simulink model "BCM2_4"  (R2021b)
settings: Solver=FixedStepDiscrete  StartTime=0.0  StopTime=1  FixedStep=0.001  RelTol=1e-3  EnableMultiTasking=on
InitFcn:
  | mbd_mpc_consistency_checks(bdroot(gcs));
model workspace (MAT data in the model file):
  CAN_rec = Simulink.Signal
  CAN_rec.DataType = 'Bus: CAN_receive'
  CAN_rec.Dimensions = 1
  CAN_rec.DimensionsMode = 'auto'
  CAN_rec.Complexity = 'auto'
  CAN_rec.SampleTime = -1
  CAN_rec.SamplingMode = 'auto'
  CAN_transm_stat = Simulink.Signal
  CAN_transm_stat.DataType = 'boolean'
  CAN_transm_stat.Dimensions = 64
  CAN_transm_stat.DimensionsMode = 'auto'
  CAN_transm_stat.Complexity = 'auto'
  CAN_transm_stat.SampleTime = -1
  CAN_transm_stat.SamplingMode = 'auto'
  CAN_trm = Simulink.Signal
  CAN_trm.DataType = 'Bus: CAN_transmit'
  CAN_trm.Dimensions = 1
  CAN_trm.DimensionsMode = 'auto'
  CAN_trm.Complexity = 'auto'
  CAN_trm.SampleTime = -1
  CAN_trm.SamplingMode = 'auto'
  DITHER_CFB0 = Simulink.Parameter
  DITHER_CFB0.DataType = 'uint32'
  DITHER_CFB0.Complexity = 'real'
  DITHER_CFB0.Dimensions = [0 0]
  DITHER_CFB1 = Simulink.Parameter
  DITHER_CFB1.DataType = 'uint32'
  DITHER_CFB1.Complexity = 'real'
  DITHER_CFB1.Dimensions = [0 0]
  DITHER_CFB2 = Simulink.Parameter
  DITHER_CFB2.DataType = 'uint32'
  DITHER_CFB2.Complexity = 'real'
  DITHER_CFB2.Dimensions = [0 0]
  DITHER_EN0 = Simulink.Parameter
  DITHER_EN0.DataType = 'uint32'
  DITHER_EN0.Complexity = 'real'
  DITHER_EN0.Dimensions = [0 0]
  DITHER_EN1 = Simulink.Parameter
  DITHER_EN1.DataType = 'uint32'
  DITHER_EN1.Complexity = 'real'
  DITHER_EN1.Dimensions = [0 0]
  DITHER_EN2 = Simulink.Parameter
  DITHER_EN2.DataType = 'uint32'
  DITHER_EN2.Complexity = 'real'
  DITHER_EN2.Dimensions = [0 0]
  DITHER_SIZE0 = Simulink.Parameter
  DITHER_SIZE0.DataType = 'uint32'
  DITHER_SIZE0.Complexity = 'real'
  DITHER_SIZE0.Dimensions = [0 0]
  DITHER_SIZE1 = Simulink.Parameter
  DITHER_SIZE1.DataType = 'uint32'
  DITHER_SIZE1.Complexity = 'real'
  DITHER_SIZE1.Dimensions = [0 0]
  DITHER_SIZE2 = Simulink.Parameter
  DITHER_SIZE2.DataType = 'uint32'
  DITHER_SIZE2.Complexity = 'real'
  DITHER_SIZE2.Dimensions = [0 0]
  DITHER_STEP0 = Simulink.Parameter
  DITHER_STEP0.DataType = 'uint32'
  DITHER_STEP0.Complexity = 'real'
  DITHER_STEP0.Dimensions = [0 0]
  DITHER_STEP1 = Simulink.Parameter
  DITHER_STEP1.DataType = 'uint32'
  DITHER_STEP1.Complexity = 'real'
  DITHER_STEP1.Dimensions = [0 0]
  DITHER_STEP2 = Simulink.Parameter
  DITHER_STEP2.DataType = 'uint32'
  DITHER_STEP2.Complexity = 'real'
  DITHER_STEP2.Dimensions = [0 0]
  DITHER_SYNC0 = Simulink.Parameter
  DITHER_SYNC0.DataType = 'uint32'
  DITHER_SYNC0.Complexity = 'real'
  DITHER_SYNC0.Dimensions = [0 0]
  DITHER_SYNC1 = Simulink.Parameter
  DITHER_SYNC1.DataType = 'uint32'
  DITHER_SYNC1.Complexity = 'real'
  DITHER_SYNC1.Dimensions = [0 0]
  DITHER_SYNC2 = Simulink.Parameter
  DITHER_SYNC2.DataType = 'uint32'
  DITHER_SYNC2.Complexity = 'real'
  DITHER_SYNC2.Dimensions = [0 0]
  ECUMbut = Simulink.Signal
  ECUMbut.DataType = 'Bus: Ecumaster_buttons'
  ECUMbut.Dimensions = 1
  ECUMbut.DimensionsMode = 'Fixed'
  ECUMbut.Complexity = 'real'
  ECUMbut.SampleTime = -1
  ECUMbut.SamplingMode = 'auto'
  FAULTN = Simulink.Signal
  FAULTN.DataType = 'boolean'
  FAULTN.Dimensions = 1
  FAULTN.DimensionsMode = 'Fixed'
  FAULTN.Complexity = 'real'
  FAULTN.SampleTime = -1
  FAULTN.SamplingMode = 'auto'
  FAULTN.InitialValue = 'false'
  FM0 = Simulink.Parameter
  FM0.DataType = 'uint32'
  FM0.Complexity = 'real'
  FM0.Dimensions = [0 0]
  FM1 = Simulink.Parameter
  FM1.DataType = 'uint32'
  FM1.Complexity = 'real'
  FM1.Dimensions = [0 0]
  FM2 = Simulink.Parameter
  FM2.DataType = 'uint32'
  FM2.Complexity = 'real'
  FM2.Dimensions = [0 0]
  FME = Simulink.Parameter
  FME.DataType = 'uint32'
  FME.Complexity = 'real'
  FME.Dimensions = [0 0]
  Fsys_M = Simulink.Parameter
  Fsys_M.DataType = 'uint32'
  Fsys_M.Complexity = 'real'
  Fsys_M.Dimensions = [0 0]
  Fsys_N = Simulink.Parameter
  Fsys_N.DataType = 'uint32'
  Fsys_N.Complexity = 'real'
  Fsys_N.Dimensions = [0 0]
  Fsys_WDEN = Simulink.Parameter
  Fsys_WDEN.DataType = 'uint32'
  Fsys_WDEN.Complexity = 'real'
  Fsys_WDEN.Dimensions = [0 0]
  Fsys_div = Simulink.Parameter
  Fsys_div.DataType = 'uint32'
  Fsys_div.Complexity = 'real'
  Fsys_div.Dimensions = [0 0]
  HL0 = Simulink.Parameter
  HL0.DataType = 'uint32'
  HL0.Complexity = 'real'
  HL0.Dimensions = [0 0]
  HL1 = Simulink.Parameter
  HL1.DataType = 'uint32'
  HL1.Complexity = 'real'
  HL1.Dimensions = [0 0]
  HL2 = Simulink.Parameter
  HL2.DataType = 'uint32'
  HL2.Complexity = 'real'
  HL2.Dimensions = [0 0]
  IDIAG0 = Simulink.Parameter
  IDIAG0.DataType = 'uint32'
  IDIAG0.Complexity = 'real'
  IDIAG0.Dimensions = [0 0]
  IDIAG1 = Simulink.Parameter
  IDIAG1.DataType = 'uint32'
  IDIAG1.Complexity = 'real'
  IDIAG1.Dimensions = [0 0]
  IDIAG2 = Simulink.Parameter
  IDIAG2.DataType = 'uint32'
  IDIAG2.Complexity = 'real'
  IDIAG2.Dimensions = [0 0]
  Ivalve = Simulink.Signal
  Ivalve.DataType = 'uint16'
  Ivalve.Dimensions = 3
  Ivalve.DimensionsMode = 'Fixed'
  Ivalve.Complexity = 'real'
  Ivalve.SampleTime = -1
  Ivalve.SamplingMode = 'auto'
  KI_index0 = Simulink.Parameter
  KI_index0.DataType = 'uint32'
  KI_index0.Complexity = 'real'
  KI_index0.Dimensions = [0 0]
  KI_index1 = Simulink.Parameter
  KI_index1.DataType = 'uint32'
  KI_index1.Complexity = 'real'
  KI_index1.Dimensions = [0 0]
  KI_index2 = Simulink.Parameter
  KI_index2.DataType = 'uint32'
  KI_index2.Complexity = 'real'
  KI_index2.Dimensions = [0 0]
  PWM_Period0 = Simulink.Parameter
  PWM_Period0.DataType = 'uint32'
  PWM_Period0.Complexity = 'real'
  PWM_Period0.Dimensions = [0 0]
  PWM_Period1 = Simulink.Parameter
  PWM_Period1.DataType = 'uint32'
  PWM_Period1.Complexity = 'real'
  PWM_Period1.Dimensions = [0 0]
  PWM_Period2 = Simulink.Parameter
  PWM_Period2.DataType = 'uint32'
  PWM_Period2.Complexity = 'real'
  PWM_Period2.Dimensions = [0 0]
  RESN = Simulink.Signal
  RESN.DataType = 'boolean'
  RESN.Dimensions = 1
  RESN.DimensionsMode = 'Fixed'
  RESN.Complexity = 'real'
  RESN.SampleTime = -1
  RESN.SamplingMode = 'auto'
  RESN.InitialValue = 'false'
  SR0 = Simulink.Parameter
  SR0.DataType = 'uint32'
  SR0.Complexity = 'real'
  SR0.Dimensions = [0 0]
  SR1 = Simulink.Parameter
  SR1.DataType = 'uint32'
  SR1.Complexity = 'real'
  SR1.Dimensions = [0 0]
  SR2 = Simulink.Parameter
  SR2.DataType = 'uint32'
  SR2.Complexity = 'real'
  SR2.Dimensions = [0 0]
  Vparam = Simulink.Signal
  Vparam.DataType = 'Bus: Vparameters'
  Vparam.Dimensions = 1
  Vparam.DimensionsMode = 'Fixed'
  Vparam.Complexity = 'real'
  Vparam.SampleTime = -1
  Vparam.SamplingMode = 'auto'
  block_tle = Simulink.Signal
  block_tle.DataType = 'boolean'
  block_tle.Dimensions = 4
  block_tle.DimensionsMode = 'auto'
  block_tle.Complexity = 'real'
  block_tle.SampleTime = -1
  block_tle.SamplingMode = 'auto'
  disp = Simulink.Signal
  disp.DataType = 'Bus: display'
  disp.Dimensions = 1
  disp.DimensionsMode = 'auto'
  disp.Complexity = 'auto'
  disp.SampleTime = -1
  disp.SamplingMode = 'auto'
  ee_adr = Simulink.Signal
  ee_adr.DataType = 'uint8'
  ee_adr.Dimensions = 1
  ee_adr.DimensionsMode = 'auto'
  ee_adr.Complexity = 'real'
  ee_adr.SampleTime = -1
  ee_adr.SamplingMode = 'auto'
  ee_en_rd = Simulink.Signal
  ee_en_rd.DataType = 'boolean'
  ee_en_rd.Dimensions = 1
  ee_en_rd.DimensionsMode = 'auto'
  ee_en_rd.Complexity = 'real'
  ee_en_rd.SampleTime = -1
  ee_en_rd.SamplingMode = 'auto'
  ee_en_wr = Simulink.Signal
  ee_en_wr.DataType = 'boolean'
  ee_en_wr.Dimensions = 1
  ee_en_wr.DimensionsMode = 'auto'
  ee_en_wr.Complexity = 'real'
  ee_en_wr.SampleTime = -1
  ee_en_wr.SamplingMode = 'auto'
  ee_idle = Simulink.Signal
  ee_idle.DataType = 'boolean'
  ee_idle.Dimensions = 1
  ee_idle.DimensionsMode = 'auto'
  ee_idle.Complexity = 'real'
  ee_idle.SampleTime = -1
  ee_idle.SamplingMode = 'auto'
  ee_read = Simulink.Signal
  ee_read.DataType = 'uint16'
  ee_read.Dimensions = 1
  ee_read.DimensionsMode = 'auto'
  ee_read.Complexity = 'real'
  ee_read.SampleTime = -1
  ee_read.SamplingMode = 'auto'
  ee_recv = Simulink.Signal
  ee_recv.DataType = 'uint8'
  ee_recv.Dimensions = [1 5]
  ee_recv.DimensionsMode = 'auto'
  ee_recv.Complexity = 'real'
  ee_recv.SampleTime = -1
  ee_recv.SamplingMode = 'auto'
  ee_send = Simulink.Signal
  ee_send.DataType = 'uint16'
  ee_send.Dimensions = 1
  ee_send.DimensionsMode = 'auto'
  ee_send.Complexity = 'real'
  ee_send.SampleTime = -1
  ee_send.SamplingMode = 'auto'
  in_stats = Simulink.Signal
  in_stats.DataType = 'Bus: inputs_stat'
  in_stats.Dimensions = 1
  in_stats.DimensionsMode = 'Fixed'
  in_stats.Complexity = 'real'
  in_stats.SampleTime = -1
  in_stats.SamplingMode = 'auto'
  inputs = Simulink.Signal
  inputs.DataType = 'boolean'
  inputs.Dimensions = 44
  inputs.DimensionsMode = 'Fixed'
  inputs.Complexity = 'real'
  inputs.SampleTime = -1
  inputs.SamplingMode = 'auto'
  light = Simulink.Signal
  light.DataType = 'Bus: light_outs'
  light.Dimensions = 1
  light.DimensionsMode = 'Fixed'
  light.Complexity = 'real'
  light.SampleTime = -1
  light.SamplingMode = 'auto'
  out_drv = Simulink.Signal
  out_drv.DataType = 'boolean'
  out_drv.Dimensions = 16
  out_drv.DimensionsMode = 'Fixed'
  out_drv.Complexity = 'real'
  out_drv.SampleTime = -1
  out_drv.SamplingMode = 'auto'
  out_drv_test = Simulink.Signal
  out_drv_test.DataType = 'boolean'
  out_drv_test.Dimensions = 16
  out_drv_test.DimensionsMode = 'Fixed'
  out_drv_test.Complexity = 'real'
  out_drv_test.SampleTime = -1
  out_drv_test.SamplingMode = 'auto'
  out_test_en = Simulink.Signal
  out_test_en.DataType = 'boolean'
  out_test_en.Dimensions = 1
  out_test_en.DimensionsMode = 'Fixed'
  out_test_en.Complexity = 'real'
  out_test_en.SampleTime = -1
  out_test_en.SamplingMode = 'auto'
  recv_spi2 = Simulink.Signal
  recv_spi2.DataType = 'uint8'
  recv_spi2.Dimensions = 8
  recv_spi2.DimensionsMode = 'Fixed'
  recv_spi2.Complexity = 'real'
  recv_spi2.SampleTime = -1
  recv_spi2.SamplingMode = 'auto'
  ret = Simulink.Signal
  ret.DataType = 'Bus: retarder'
  ret.Dimensions = 1
  ret.DimensionsMode = 'Fixed'
  ret.Complexity = 'real'
  ret.SampleTime = -1
  ret.SamplingMode = 'auto'
  spi_rcv_tle82453 = Simulink.Signal
  spi_rcv_tle82453.DataType = 'uint8'
  spi_rcv_tle82453.Dimensions = [1 4]
  spi_rcv_tle82453.DimensionsMode = 'auto'
  spi_rcv_tle82453.Complexity = 'real'
  spi_rcv_tle82453.SampleTime = -1
  spi_rcv_tle82453.SamplingMode = 'auto'
  tle82453_Ivlv = Simulink.Signal
  tle82453_Ivlv.DataType = 'uint8'
  tle82453_Ivlv.Dimensions = 3
  tle82453_Ivlv.DimensionsMode = 'auto'
  tle82453_Ivlv.Complexity = 'real'
  tle82453_Ivlv.SampleTime = -1
  tle82453_Ivlv.SamplingMode = 'auto'
  tle82453_Ivlv.InitialValue = '[0 0 0]'
  tle82453_err = Simulink.Signal
  tle82453_err.DataType = 'uint32'
  tle82453_err.Dimensions = 1
  tle82453_err.DimensionsMode = 'auto'
  tle82453_err.Complexity = 'real'
  tle82453_err.SampleTime = -1
  tle82453_err.SamplingMode = 'auto'
  tle82453_reset = Simulink.Signal
  tle82453_reset.DataType = 'boolean'
  tle82453_reset.Dimensions = 1
  tle82453_reset.DimensionsMode = 'Fixed'
  tle82453_reset.Complexity = 'real'
  tle82453_reset.SampleTime = -1
  tle82453_reset.SamplingMode = 'auto'
  tle82453_reset.InitialValue = '0'
  wtdg_CAN = Simulink.Signal
  wtdg_CAN.DataType = 'Bus: WTDG_CAN'
  wtdg_CAN.Dimensions = 1
  wtdg_CAN.DimensionsMode = 'auto'
  wtdg_CAN.Complexity = 'real'
  wtdg_CAN.SampleTime = -1
  wtdg_CAN.SamplingMode = 'auto'
undefined symbols (not defined in the file or in its folder): color, LQFP
libraries: simulink x68, mbd_mpc574x_ec_toolbox x50, canmsglib x42, hdlsllib x9, commutil2 x7, etargetslib x4
(part 1 of 6)
Description:
  | Блок управления BCM
  | В качестве драйвера входов используется MC33978
settings Model: Creator=Дешкин Е.А.  LastModifiedBy=km-gir
settings SolverCC: AlgebraicLoopSolver=TrustRegion  AutoInsertRateTranBlk=on
settings DataIOCC: ExternalInput=off  InitialState=off  LimitDataPoints=on  SaveFormat=Array  SaveOutput=off  SignalLogging=off  SaveTime=off  ReturnWorkspaceOutputs=off
settings OptimizationCC: DefaultParameterBehavior=Inlined  PassReuseOutputArgsAs=Individual arguments  LifeSpan=inf  EfficientTunableParamExpr=on
settings DebuggingCC: MergeDetectMultiDrivingBlocksExec=none  SolverPrmCheckMsg=warning  InheritedTsInSrcMsg=none  MultiTaskDSMMsg=none  SingleTaskRateTransMsg=error  ParameterTunabilityLossMsg=error  UnconnectedInputMsg=error  UnconnectedOutputMsg=error  UnconnectedLineMsg=error  AllowSymbolicDim=off  UnknownTsInhSupMsg=error  StateNameClashWarn=warning  SFUnexpectedBacktrackingDiag=warning  SFNoUnconditionalDefaultTransitionDiag=warning  SFMachineParentedDataDiag=warning  ArithmeticOperatorsInVariantConditions=warning
settings HardwareCC: ProdBitPerPointer=32  ProdBitPerSizeT=32  ProdBitPerPtrDiffT=32  ProdLargestAtomicInteger=Long  ProdLargestAtomicFloat=Double  ProdEndianess=BigEndian  ProdWordSize=32  ProdHWDeviceType=Motorola PowerPC
settings ModelReferenceCC: PropagateSignalLabelsOutOfModel=off
settings SFSimCC: SimUseLocalCustomCode=off  MATLABDynamicMemAlloc=off  CustomCodeUndefinedFunction=UseInterfaceOnly
settings RTWCC: Description=Model Based Design Toolbox MPC57xx Code Generation Target  SystemTargetFile=mbd_mpc574x.tlc  MakeCommand=mbd_mpc574x_make_rtw  TemplateMakefile=mbd_mpc574x.tmf  GenerateReport=on  RTWUseLocalCustomCode=off  IncludeHyperlinkInReport=on  LaunchReport=on  GenerateTraceInfo=on  GenerateTraceReport=on  GenerateTraceReportSl=on  GenerateTraceReportSf=on  GenerateTraceReportEml=on
settings CodeAppCC: ForceParamTrailComments=on  IgnoreCustomStorageClasses=off  OperatorAnnotations=on  SimulinkDataObjDesc=on  SFDataObjDesc=on  MATLABFcnDesc=on  InsertBlockDesc=on  StateflowObjectComments=on  MATLABSourceComments=on
settings STFCustomTargetCC: MultiwordLength=256  CombineOutputUpdateFcns=on  ERTCustomFileBanners=on  SupportContinuousTime=off  SupportNonInlinedSFcns=off  RemoveResetFunc=on  MATLABClassNameForMDSCustomization=Simulink.SoftwareTarget.ERTCustomization  GRTInterface=off  SystemTargetFile=mbd_mpc574x.tlc
settings ERTTargetCC: ParMdlRefBuildCompliant=off  CompOptLevelCompliant=off  ConcurrentExecutionCompliant=off  ModelStepFunctionPrototypeControlCompliant=off  CPPClassGenCompliant=off  UseToolchainInfoCompliant=off  InlinedParameterPlacement=NonHierarchical  ERTSrcFileBannerTemplate=mbd_ert_code_template.cgt  ERTHdrFileBannerTemplate=mbd_ert_code_template.cgt  ERTDataSrcFileTemplate=mbd_ert_code_template.cgt  ERTDataHdrFileTemplate=mbd_ert_code_template.cgt  ERTCustomFileTemplate=example_file_process.tlc
settings ConfigComp: CovMetricSettings=dw  CovSaveCumulativeToWorkspaceVar=on  CovSaveSingleToWorkspaceVar=on  CovExternalEMLEnable=off

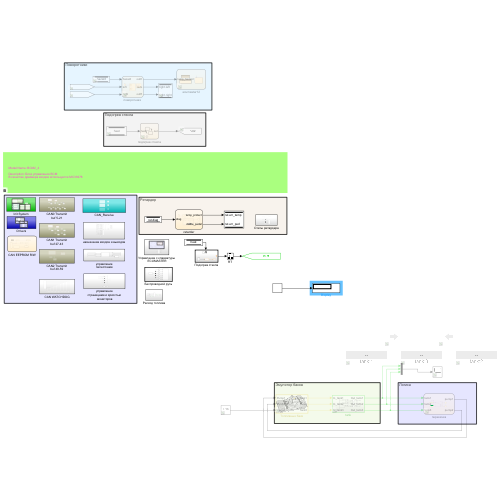
[thumbnail: Simulink's stored preview of the top-level diagram]
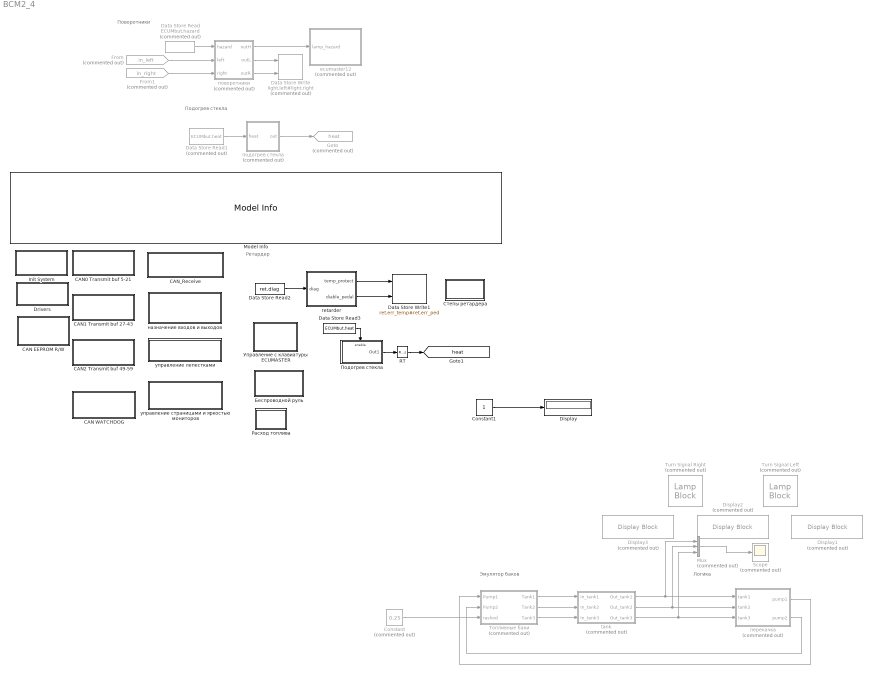
== system BCM2_4 ==
  note: Логика
  note: Эмулятор баков
  note: Подогрев стекла
  note: Поворотники
  note: Ретардер
  CAN EEPROM R/W : Stateflow chart  TreatAsAtomicUnit=on
  CAN WATCHDOG : Subsystem
  CAN0 Transmit buf 5-21 : Subsystem
  CAN1 Transmit buf 27-43 : Subsystem
  CAN2 Transmit buf 49-59 : Subsystem
  CAN_Receive : Subsystem  Priority=2
  Constant : Constant  Commented=on  Value=0.25
  Constant1 : Constant
  Data Store Read : DataStoreRead  Commented=on  DataStoreName=ECUMbut  DataStoreElements=ECUMbut.hazard  IndexOptions=Index vector (dialog)  Indices=1  OutputSizes=1
  Data Store Read1 : DataStoreRead  Commented=on  DataStoreName=ECUMbut  DataStoreElements=ECUMbut.heat  IndexOptions=Index vector (dialog)  Indices=1  OutputSizes=1
  Data Store Read2 : DataStoreRead  DataStoreName=ret  DataStoreElements=ret.diag  IndexOptions=Index vector (dialog)  Indices=1  OutputSizes=1
  Data Store Read3 : DataStoreRead  DataStoreName=ECUMbut  DataStoreElements=ECUMbut.heat  IndexOptions=Index vector (dialog)  Indices=1  OutputSizes=1
  Data Store Write : DataStoreWrite  Commented=on  DataStoreName=light  DataStoreElements=light.left#light.right  IndexOptions=Index vector (dialog)  Indices=1  OutputSizes=1
  Data Store Write1 : DataStoreWrite  DataStoreName=ret  DataStoreElements=ret.err_temp#ret.err_ped  IndexOptions=Index vector (dialog)  Indices=1  OutputSizes=1
  Display : Display
  Display1 : DisplayBlock  Commented=on  LabelPosition=Bottom  Format=short  Transparency=1
  Display2 : DisplayBlock  Commented=on  LabelPosition=Bottom  Format=short  Transparency=1
  Display3 : DisplayBlock  Commented=on  LabelPosition=Bottom  Format=short  Transparency=1
  Drivers : Subsystem
  From : From  Commented=on  GotoTag=in_left  TagVisibility=global
  From1 : From  Commented=on  GotoTag=in_right  TagVisibility=global
  Goto : Goto  Commented=on  GotoTag=heat  TagVisibility=global
  Init System : Subsystem
  Model Info : simulink/Model-Wide Utilities/Model Info  Frame=off  DisplayStringWithTags=|  HorizontalTextAlignment=Left  LeftAlignmentValue=0.02
      | Model Name: %<ModelName>
      | 
      | Description: %<Description>
  Mux : Mux  Commented=on  Inputs=3
  RT : RateTransition  OutPortSampleTime=0.01
  Scope : Scope  Commented=on
  Turn Signal Left : LampBlock  Commented=on  LabelPosition=Hide  Icon=TurnSignalLeft
  Turn Signal Right : LampBlock  Commented=on  LabelPosition=Hide  Icon=TurnSignalRight
  ecumaster12 : Stateflow chart  Commented=on  TreatAsAtomicUnit=on
  retarder : Stateflow chart  TreatAsAtomicUnit=on
  tank : Subsystem  Commented=on
  Беспроводной руль : Subsystem  TreatAsAtomicUnit=on  SystemSampleTime=0.01
  Подогрев стекла : Subsystem  TreatAsAtomicUnit=on
  Расход топлива : Subsystem
  Степы ретардера : Subsystem
  Топливные баки : Subsystem  Commented=on  TreatAsAtomicUnit=on  SystemSampleTime=1  mask{ft1=290, ft2=230, ft3=50}
      mask prompts: ft1 "Fuel tank1"; ft2 "Fuel tank2"; ft3 "Fuel tank3"
      mask Display: image('$imagefile'); % Use "Edit Image" on toolstrip to change.
  Управление с клавиатуры ECUMASTER : Subsystem
  назначение входов и выходов : Subsystem
  перекачка : Stateflow chart  Commented=on  TreatAsAtomicUnit=on
  поворотники : Stateflow chart  Commented=on  TreatAsAtomicUnit=on
  подогрев стекла : Stateflow chart  Commented=on  TreatAsAtomicUnit=on  mask{heat_off=3, heat_on=6}
      mask prompts: heat_off "Time OFF, minutes"; heat_on "Time ON, minutes"
  управление лепестками : Subsystem
  управление страницами и яркостью мониторов : Subsystem
  tag scope: heat=global
  wires:
  Data Store Read/1 -> поворотники/1(hazard)
  From/1 -> поворотники/2(left)
  From1/1 -> поворотники/3(right)
  поворотники/1(outH) -> ecumaster12/1(lamp_hazard)
  подогрев стекла/1(out) -> Goto/1
  поворотники/2(outL) -> Data Store Write/1
  поворотники/3(outR) -> Data Store Write/2
  retarder/2(" diable_pedal") -> Data Store Write1/2
  retarder/1(" temp_protect") -> Data Store Write1/1
  Data Store Read2/1 -> retarder/1(diag)
  Data Store Read1/1 -> подогрев стекла/1(heat)
  RT/1 -> [heat]
  Data Store Read3/1 -> Подогрев стекла/Enable
  Подогрев стекла/1(Out1) -> RT/1
  Топливные баки/1(Tank1) -> tank/1(In_tank1)
  Топливные баки/2(Tank2) -> tank/2(In_tank2)
  Топливные баки/3(Tank3) -> tank/3(In_tank3)
  tank/1(Out_tank1) -> Mux/1, перекачка/1(tank1)
  tank/2(Out_tank2) -> Mux/2, перекачка/2(tank2)
  tank/3(Out_tank3) -> Mux/3, перекачка/3(tank3)
  перекачка/2(pump2) -> Топливные баки/2(Pump2)
  Mux/1 -> Scope/1
  Constant/1 -> Топливные баки/3(rashod)
  перекачка/1(pump1) -> Топливные баки/1(Pump1)
  Constant1/1 -> Display/1

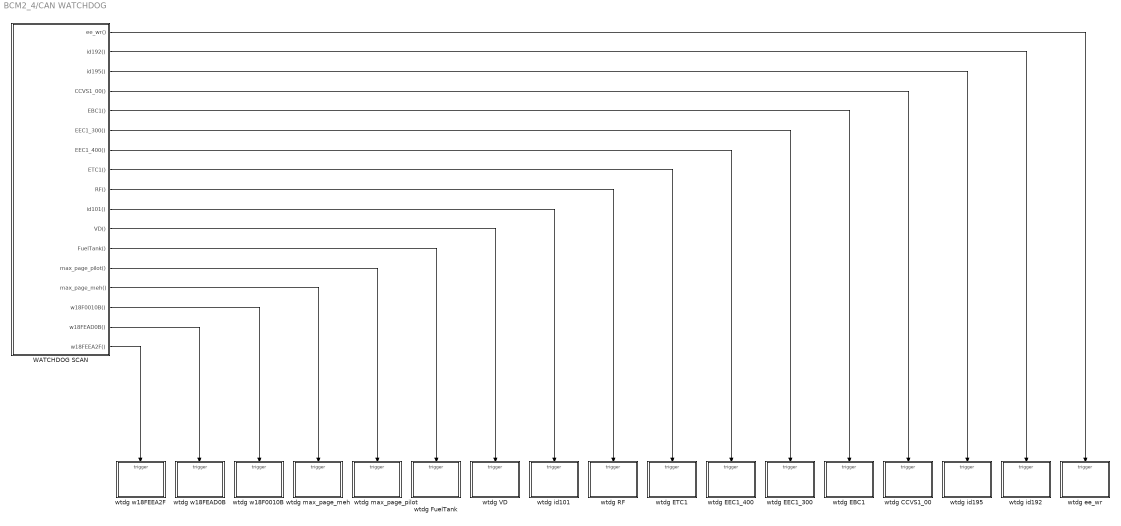
== system BCM2_4/CAN WATCHDOG ==
  WATCHDOG SCAN : Stateflow chart  TreatAsAtomicUnit=on
  wtdg CCVS1_00 : Subsystem  TreatAsAtomicUnit=on
  wtdg EBC1 : Subsystem  TreatAsAtomicUnit=on
  wtdg EEC1_300 : Subsystem  TreatAsAtomicUnit=on
  wtdg EEC1_400 : Subsystem  TreatAsAtomicUnit=on
  wtdg ETC1 : Subsystem  TreatAsAtomicUnit=on
  wtdg FuelTank : Subsystem  TreatAsAtomicUnit=on
  wtdg RF : Subsystem  TreatAsAtomicUnit=on
  wtdg VD : Subsystem  TreatAsAtomicUnit=on
  wtdg ee_wr : Subsystem  TreatAsAtomicUnit=on
  wtdg id101 : Subsystem  TreatAsAtomicUnit=on
  wtdg id192 : Subsystem  TreatAsAtomicUnit=on
  wtdg id195 : Subsystem  TreatAsAtomicUnit=on
  wtdg max_page_meh : Subsystem  TreatAsAtomicUnit=on
  wtdg max_page_pilot : Subsystem  TreatAsAtomicUnit=on
  wtdg w18F0010B : Subsystem  TreatAsAtomicUnit=on
  wtdg w18FEAD0B : Subsystem  TreatAsAtomicUnit=on
  wtdg w18FEEA2F : Subsystem  TreatAsAtomicUnit=on
  wires:
  WATCHDOG SCAN/9(RF()) -> wtdg RF/Trigger
  WATCHDOG SCAN/8(ETC1()) -> wtdg ETC1/Trigger
  WATCHDOG SCAN/7(EEC1_400()) -> wtdg EEC1_400/Trigger
  WATCHDOG SCAN/6(EEC1_300()) -> wtdg EEC1_300/Trigger
  WATCHDOG SCAN/5(EBC1()) -> wtdg EBC1/Trigger
  WATCHDOG SCAN/4(CCVS1_00()) -> wtdg CCVS1_00/Trigger
  WATCHDOG SCAN/3(id195()) -> wtdg id195/Trigger
  WATCHDOG SCAN/2(id192()) -> wtdg id192/Trigger
  WATCHDOG SCAN/1(ee_wr()) -> wtdg ee_wr/Trigger
  WATCHDOG SCAN/10(id101()) -> wtdg id101/Trigger
  WATCHDOG SCAN/11(VD()) -> wtdg VD/Trigger
  WATCHDOG SCAN/12(FuelTank()) -> wtdg FuelTank/Trigger
  WATCHDOG SCAN/13(max_page_pilot()) -> wtdg max_page_pilot/Trigger
  WATCHDOG SCAN/14(max_page_meh()) -> wtdg max_page_meh/Trigger
  WATCHDOG SCAN/15(w18F0010B()) -> wtdg w18F0010B/Trigger
  WATCHDOG SCAN/16(w18FEAD0B()) -> wtdg w18FEAD0B/Trigger
  WATCHDOG SCAN/17(w18FEEA2F()) -> wtdg w18FEEA2F/Trigger

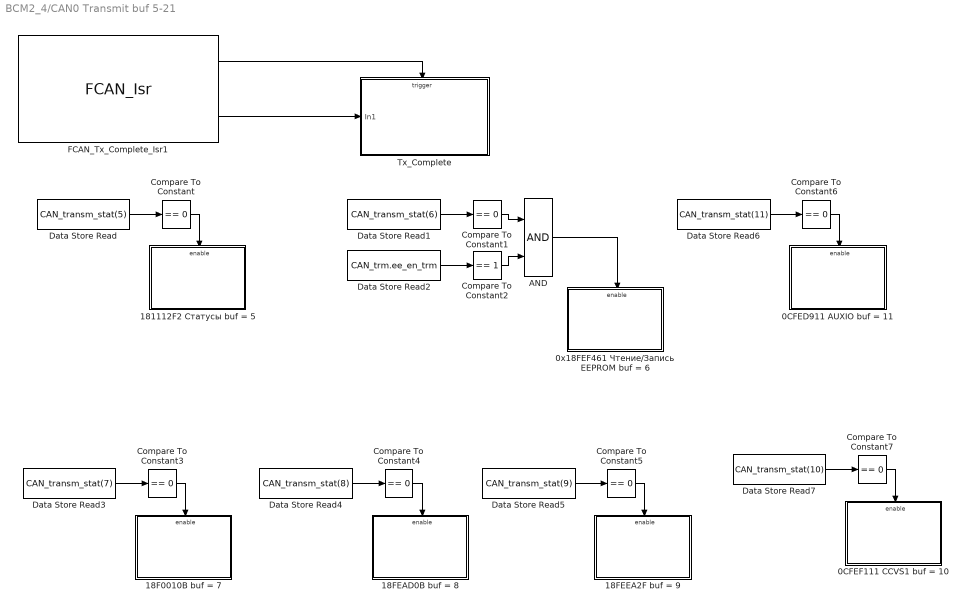
== system BCM2_4/CAN0 Transmit buf 5-21 ==
  0CFED911 AUXIO buf = 11 : Subsystem
  0CFEF111 CCVS1 buf = 10 : Subsystem
  0x18FEF461 Чтение/Запись EEPROM buf = 6 : Subsystem
  181112F2 Статусы buf = 5 : Subsystem
  18F0010B buf = 7 : Subsystem
  18FEAD0B buf = 8 : Subsystem
  18FEEA2F buf = 9 : Subsystem
  AND : Logic  IconShape=distinctive  AllPortsSameDT=off  OutDataTypeStr=boolean
  Compare To Constant{,1,3..7} (7 alike) : simulink/Logic and Bit Operations/Compare To Constant  relop===  const=0  OutDataTypeStr=boolean
  Compare To Constant2 : simulink/Logic and Bit Operations/Compare To Constant  relop===  const=1  OutDataTypeStr=boolean
  Data Store Read : DataStoreRead  DataStoreName=CAN_transm_stat  DataStoreElements=CAN_transm_stat(5)  IndexOptions=Index vector (dialog)  Indices=1  OutputSizes=1
  Data Store Read1 : DataStoreRead  DataStoreName=CAN_transm_stat  DataStoreElements=CAN_transm_stat(6)  IndexOptions=Index vector (dialog)  Indices=1  OutputSizes=1
  Data Store Read2 : DataStoreRead  DataStoreName=CAN_trm  DataStoreElements=CAN_trm.ee_en_trm  IndexOptions=Index vector (dialog)  Indices=1  OutputSizes=1
  Data Store Read3 : DataStoreRead  DataStoreName=CAN_transm_stat  DataStoreElements=CAN_transm_stat(7)  IndexOptions=Index vector (dialog)  Indices=1  OutputSizes=1
  Data Store Read4 : DataStoreRead  DataStoreName=CAN_transm_stat  DataStoreElements=CAN_transm_stat(8)  IndexOptions=Index vector (dialog)  Indices=1  OutputSizes=1
  Data Store Read5 : DataStoreRead  DataStoreName=CAN_transm_stat  DataStoreElements=CAN_transm_stat(9)  IndexOptions=Index vector (dialog)  Indices=1  OutputSizes=1
  Data Store Read6 : DataStoreRead  DataStoreName=CAN_transm_stat  DataStoreElements=CAN_transm_stat(11)  IndexOptions=Index vector (dialog)  Indices=1  OutputSizes=1
  Data Store Read7 : DataStoreRead  DataStoreName=CAN_transm_stat  DataStoreElements=CAN_transm_stat(10)  IndexOptions=Index vector (dialog)  Indices=1  OutputSizes=1
  FCAN_Tx_Complete_Isr1 : mbd_mpc574x_ec_toolbox/Communication Blocks/CAN Blocks/FCAN_Isr  can_instance=0  can_event=Tx Complete
      settings: SourceProductName=NXP Model-Based Design Toolbox for MPC57xx MCUs
  Tx_Complete : Subsystem  TreatAsAtomicUnit=on
      settings: RTWSystemCode=Nonreusable function
  wires:
  FCAN_Tx_Complete_Isr1/2 -> Tx_Complete/1(In1)
  Data Store Read/1 -> Compare To Constant/1
  FCAN_Tx_Complete_Isr1/1 -> Tx_Complete/Trigger
  Compare To Constant/1 -> 181112F2 Статусы buf = 5/Enable
  AND/1 -> 0x18FEF461 Чтение/Запись EEPROM buf = 6/Enable
  Data Store Read1/1 -> Compare To Constant1/1
  Data Store Read2/1 -> Compare To Constant2/1
  Compare To Constant1/1 -> AND/1
  Compare To Constant2/1 -> AND/2
  Compare To Constant3/1 -> 18F0010B buf = 7/Enable
  Data Store Read3/1 -> Compare To Constant3/1
  Data Store Read4/1 -> Compare To Constant4/1
  Compare To Constant4/1 -> 18FEAD0B buf = 8/Enable
  Compare To Constant5/1 -> 18FEEA2F buf = 9/Enable
  Data Store Read5/1 -> Compare To Constant5/1
  Compare To Constant6/1 -> 0CFED911 AUXIO buf = 11/Enable
  Data Store Read6/1 -> Compare To Constant6/1
  Data Store Read7/1 -> Compare To Constant7/1
  Compare To Constant7/1 -> 0CFEF111 CCVS1 buf = 10/Enable

== system BCM2_4/CAN1 Transmit buf 27-43 ==
  Compare To Constant{,1..4} (5 alike) : simulink/Logic and Bit Operations/Compare To Constant  relop===  const=0  OutDataTypeStr=boolean
  Data Store Read : DataStoreRead  DataStoreName=CAN_transm_stat  DataStoreElements=CAN_transm_stat(27)  IndexOptions=Index vector (dialog)  Indices=1  OutputSizes=1
  Data Store Read1 : DataStoreRead  DataStoreName=CAN_transm_stat  DataStoreElements=CAN_transm_stat(28)  IndexOptions=Index vector (dialog)  Indices=1  OutputSizes=1
  Data Store Read2 : DataStoreRead  DataStoreName=CAN_transm_stat  DataStoreElements=CAN_transm_stat(29)  IndexOptions=Index vector (dialog)  Indices=1  OutputSizes=1
  Data Store Read3 : DataStoreRead  DataStoreName=CAN_transm_stat  DataStoreElements=CAN_transm_stat(31)  IndexOptions=Index vector (dialog)  Indices=1  OutputSizes=1
  Data Store Read4 : DataStoreRead  DataStoreName=CAN_transm_stat  DataStoreElements=CAN_transm_stat(30)  IndexOptions=Index vector (dialog)  Indices=1  OutputSizes=1
  FCAN_Tx_Complete_Isr1 : mbd_mpc574x_ec_toolbox/Communication Blocks/CAN Blocks/FCAN_Isr  can_instance=1  can_event=Tx Complete
      settings: SourceProductName=NXP Model-Based Design Toolbox for MPC57xx MCUs
  Tx_Complete : Subsystem  TreatAsAtomicUnit=on
      settings: RTWSystemCode=Nonreusable function
  Активация клавиатуры buf = 27 : Subsystem
  Цвет клавиатуры 12 buf = 28 : Subsystem
  Цвет клавиатуры 4 buf = 30 : Subsystem
  подсветка клавиатуры buf = 29 : Subsystem
  подсветка клавиатуры buf = 31 : Subsystem
  wires:
  Compare To Constant/1 -> Активация клавиатуры buf = 27/Enable
  FCAN_Tx_Complete_Isr1/1 -> Tx_Complete/Trigger
  Data Store Read/1 -> Compare To Constant/1
  FCAN_Tx_Complete_Isr1/2 -> Tx_Complete/1(In1)
  Data Store Read1/1 -> Compare To Constant1/1
  Compare To Constant1/1 -> Цвет клавиатуры 12 buf = 28/Enable
  Compare To Constant2/1 -> подсветка клавиатуры buf = 29/Enable
  Data Store Read2/1 -> Compare To Constant2/1
  Compare To Constant3/1 -> Цвет клавиатуры 4 buf = 30/Enable
  Data Store Read4/1 -> Compare To Constant3/1
  Data Store Read3/1 -> Compare To Constant4/1
  Compare To Constant4/1 -> подсветка клавиатуры buf = 31/Enable

== system BCM2_4/CAN2 Transmit buf 49-59 ==
  Compare To Constant : simulink/Logic and Bit Operations/Compare To Constant  Commented=on  relop===  const=0  OutDataTypeStr=boolean
  Data Store Read : DataStoreRead  Commented=on  DataStoreName=CAN_transm_stat  DataStoreElements=CAN_transm_stat(9)  IndexOptions=Index vector (dialog)  Indices=1  OutputSizes=1
  EBC1 0x18F0010D Педаль тормоза buf = 9 : Subsystem  Commented=on
  FCAN_Tx_Complete_Isr1 : mbd_mpc574x_ec_toolbox/Communication Blocks/CAN Blocks/FCAN_Isr  Commented=on  can_instance=2  can_event=Tx Complete
      settings: SourceProductName=NXP Model-Based Design Toolbox for MPC57xx MCUs
  Tx_Complete : Subsystem  Commented=on  TreatAsAtomicUnit=on
      settings: RTWSystemCode=Nonreusable function
  wires:
  FCAN_Tx_Complete_Isr1/2 -> Tx_Complete/1(In1)
  Data Store Read/1 -> Compare To Constant/1
  FCAN_Tx_Complete_Isr1/1 -> Tx_Complete/Trigger
  Compare To Constant/1 -> EBC1 0x18F0010D Педаль тормоза buf = 9/Enable

== system BCM2_4/CAN_Receive ==
  FCAN_Rx_Complete_Isr : mbd_mpc574x_ec_toolbox/Communication Blocks/CAN Blocks/FCAN_Isr  can_instance=0  can_event=Rx Complete
      settings: SourceProductName=NXP Model-Based Design Toolbox for MPC57xx MCUs
  FCAN_Rx_Complete_Isr1 : mbd_mpc574x_ec_toolbox/Communication Blocks/CAN Blocks/FCAN_Isr  can_instance=1  can_event=Rx Complete
      settings: SourceProductName=NXP Model-Based Design Toolbox for MPC57xx MCUs
  FCAN_Rx_Complete_Isr2 : mbd_mpc574x_ec_toolbox/Communication Blocks/CAN Blocks/FCAN_Isr  Commented=on  can_instance=2  can_event=Rx Complete
      settings: SourceProductName=NXP Model-Based Design Toolbox for MPC57xx MCUs
  RX_FIFO_Complete_Event buf 0-4 : Subsystem  TreatAsAtomicUnit=on
      settings: RTWSystemCode=Nonreusable function
  RX_FIFO_Complete_Event2 buf 22-26 : Subsystem  TreatAsAtomicUnit=on
      settings: RTWSystemCode=Nonreusable function
  RX_FIFO_Complete_Event3 buf 44-48 : Subsystem  Commented=on  TreatAsAtomicUnit=on
      settings: RTWSystemCode=Nonreusable function
  Terminator{,1,3..4} (4 alike) : Terminator
  Terminator2 : Terminator  Commented=on
  Terminator5 : Terminator  Commented=on
  wires:
  FCAN_Rx_Complete_Isr/4 -> RX_FIFO_Complete_Event buf 0-4/3(Data)
  FCAN_Rx_Complete_Isr1/4 -> RX_FIFO_Complete_Event2 buf 22-26/3(Data)
  FCAN_Rx_Complete_Isr/3 -> RX_FIFO_Complete_Event buf 0-4/2(ID)
  FCAN_Rx_Complete_Isr/5 -> Terminator/1
  FCAN_Rx_Complete_Isr1/1 -> RX_FIFO_Complete_Event2 buf 22-26/Trigger
  FCAN_Rx_Complete_Isr/6 -> Terminator1/1
  FCAN_Rx_Complete_Isr1/2 -> RX_FIFO_Complete_Event2 buf 22-26/1(MB_index)
  FCAN_Rx_Complete_Isr1/6 -> Terminator4/1
  FCAN_Rx_Complete_Isr1/5 -> Terminator3/1
  FCAN_Rx_Complete_Isr/1 -> RX_FIFO_Complete_Event buf 0-4/Trigger
  FCAN_Rx_Complete_Isr1/3 -> RX_FIFO_Complete_Event2 buf 22-26/2(ID)
  FCAN_Rx_Complete_Isr/2 -> RX_FIFO_Complete_Event buf 0-4/1(MB_index)
  FCAN_Rx_Complete_Isr2/3 -> RX_FIFO_Complete_Event3 buf 44-48/2(ID)
  FCAN_Rx_Complete_Isr2/5 -> Terminator2/1
  FCAN_Rx_Complete_Isr2/6 -> Terminator5/1
  FCAN_Rx_Complete_Isr2/2 -> RX_FIFO_Complete_Event3 buf 44-48/1(MB_index)
  FCAN_Rx_Complete_Isr2/1 -> RX_FIFO_Complete_Event3 buf 44-48/Trigger
  FCAN_Rx_Complete_Isr2/4 -> RX_FIFO_Complete_Event3 buf 44-48/3(Data)

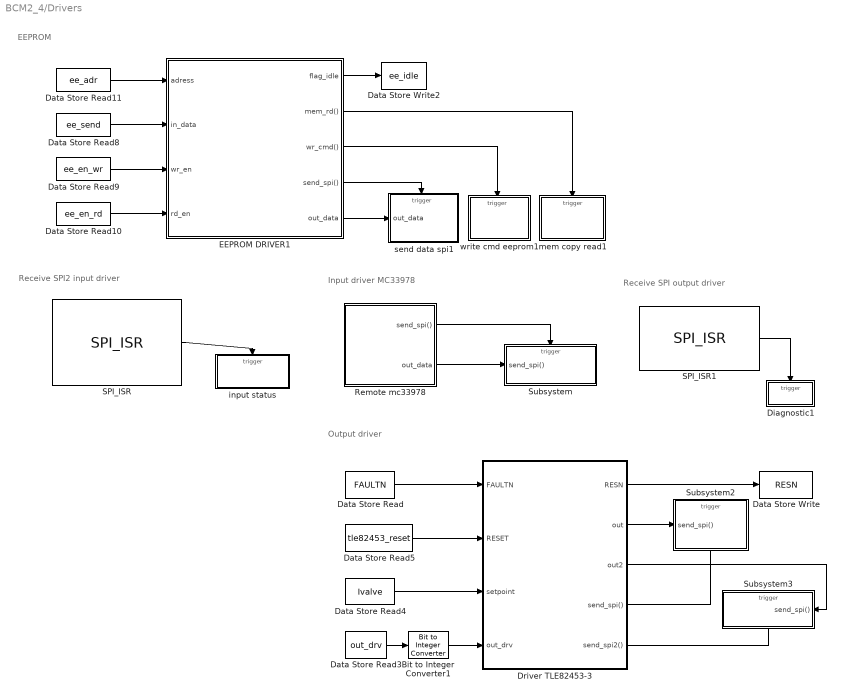
== system BCM2_4/Drivers ==
  note: Output driver
  note: Input driver MC33978
  note: Receive SPI2 input driver
  note: Receive SPI output driver
  note: EEPROM
  Bit to Integer Converter1 : commutil2/Bit to Integer Converter  nbits=16  bitOrder=LSB first  signedOutputValues=Unsigned  outDtype=uint16  outDtypeSigned=Inherit via internal rule
  Data Store Read : DataStoreRead  DataStoreName=FAULTN  IndexOptions=Index vector (dialog)  Indices=1  OutputSizes=1
  Data Store Read10 : DataStoreRead  DataStoreName=ee_en_rd  IndexOptions=Index vector (dialog)  Indices=1  OutputSizes=1
  Data Store Read11 : DataStoreRead  DataStoreName=ee_adr  IndexOptions=Index vector (dialog)  Indices=1  OutputSizes=1
  Data Store Read3 : DataStoreRead  DataStoreName=out_drv  IndexOptions=Index vector (dialog)  Indices=1  OutputSizes=1
  Data Store Read4 : DataStoreRead  DataStoreName=Ivalve  IndexOptions=Index vector (dialog)  Indices=1  OutputSizes=1
  Data Store Read5 : DataStoreRead  DataStoreName=tle82453_reset  IndexOptions=Index vector (dialog)  Indices=1  OutputSizes=1
  Data Store Read8 : DataStoreRead  DataStoreName=ee_send  IndexOptions=Index vector (dialog)  Indices=1  OutputSizes=1
  Data Store Read9 : DataStoreRead  DataStoreName=ee_en_wr  IndexOptions=Index vector (dialog)  Indices=1  OutputSizes=1
  Data Store Write : DataStoreWrite  DataStoreName=RESN  IndexOptions=Index vector (dialog)  Indices=1  OutputSizes=1
  Data Store Write2 : DataStoreWrite  DataStoreName=ee_idle  IndexOptions=Index vector (dialog)  Indices=1  OutputSizes=1
  Diagnostic1 : Subsystem
  Driver TLE82453-3 : Stateflow chart  TreatAsAtomicUnit=on  mask{Fsys_WDEN=on, Fsys_M=24, Fsys_N=5, Fsys_div=2, FME=FAULTN pin is driven low if the EN pin is low., IDIAG0=Low-Side current source is active, SR0=Set the channel slew rate to SR0 (Reset value), FM0=Channel faults do not influence the FAULTN pin (Reset value), HL0=Highside configuration, IDIAG1=Low-Side current source is active, SR1=Set the channel slew rate to SR0 (Reset value), FM1=Channel faults do not influence the FAULTN pin (Reset value), HL1=Highside configuration, IDIAG2=Low-Side current source is active, SR2=Set the channel slew rate to SR0 (Reset value), FM2=Channel faults do not influence the FAULTN pin (Reset value), HL2=Highside configuration, KI_index0=4, PWM_Period0=32, KI_index1=4, PWM_Period1=32, KI_index2=4, PWM_Period2=32, DITHER_EN0=off, DITHER_SYNC0=on, DITHER_CFB0=off, DITHER_STEP0=2, DITHER_SIZE0=55, DITHER_EN1=off, DITHER_SYNC1=on, DITHER_CFB1=off, DITHER_STEP1=2, DITHER_SIZE1=55, DITHER_EN2=off, DITHER_SYNC2=on, DITHER_CFB2=off, DITHER_STEP2=2, DITHER_SIZE2=55}
      mask prompts: Fsys_WDEN "WDEN"; Fsys_M "M"; Fsys_N "N"; IDIAG0 "IDIAG"; SR0 "SR"; FM0 "FM"; HL0 "HL"; IDIAG1 "IDIAG"; SR1 "SR"; FM1 "FM"; HL1 "HL"; IDIAG2 "IDIAG"; SR2 "SR"; FM2 "FM"; HL2 "HL"; KI_index0 "KI index"; PWM_Period0 "PWM Period"; KI_index1 "KI index"; PWM_Period1 "PWM Period"; KI_index2 "KI index"; PWM_Period2 "PWM Period"; DITHER_EN0 "EN"; DITHER_SYNC0 "SYNC"; DITHER_CFB0 "CFB MODE"; DITHER_STEP0 "Steps"; DITHER_SIZE0 "Step Size"; DITHER_EN1 "EN"; DITHER_SYNC1 "SYNC"; DITHER_CFB1 "CFB MODE"; DITHER_STEP1 "Steps"; DITHER_SIZE1 "Step Size"; DITHER_EN2 "EN"; DITHER_SYNC2 "SYNC"; DITHER_CFB2 "CFB MODE"; DITHER_STEP2 "Steps"; DITHER_SIZE2 "Step Size"
  EEPROM DRIVER1 : Stateflow chart  TreatAsAtomicUnit=on
      settings: PortSchema="{\"entries\":[{\"content\":{\"sides\":[{\"content\":{\"connectorIds\":[\"In1\",\"In3\",\"In2\",\"In4\"]},\"type\":\"ConnectorPlacement.EquallySpacedRectSide\",\"uuid\":\"5cab7dbc-4f34-4bc1-84f4-c58c6d9df884\"},{\"content\":{\"connectorIds\":[\"Out2\",\"Out5\",\"Out3\",\"Out4\",\"Out1\"],\"side\":\"RIGHT\"},\"type\":\"ConnectorPlacement.EquallySpacedRectSide\",\"uuid\":\"1fd58a09-6a45-4f4a-8662-21037d1a1ead\"},{\"content\":{\"connectorIds\":[],\"side\":\"TOP\"},\"type\":\"ConnectorPlacement.EquallySpacedRectSide\",\"uuid\":\"9b2b79a4-3bc8-4a10-b70e-6560a0b04ba0\"},{\"content\":{\"connectorIds\":[],\"side\":\"HIDDEN\"},\"type\":\"ConnectorPlacement.EquallySpacedRectSide\",\"uuid\":\"946031be-3090-4ce2-8ebf-61eb7e674520\"}]},\"type\":\"ConnectorPlacement.EquallySpacedConnector\",\"uuid\":\"3fd12340-b8f6-4bc7-a994-8b1af25b216c\"}],\"packageUris\":[\"http://schema.mathworks.com/mf0/Connector/R2020b\"],\"version\":\"1.0\"}"
  Remote mc33978 : Stateflow chart  mask{in_bl1=off, in_bl2=off, in_bl3=off, in_bl4=off, in_bl5=off, in_bl6=off, in_bl7=off, in_bl8=off, in_bl9=off, in_bl10=off, in_bl11=off, in_bl12=off, in_bl13=off, in_bl14=off, in_bl15=off, in_bl16=off}
      settings: PortSchema="{\"entries\":[{\"content\":{\"sides\":[{\"content\":{\"connectorIds\":[]},\"type\":\"ConnectorPlacement.EquallySpacedRectSide\",\"uuid\":\"74b2e3f0-d8be-4163-9148-af4954deab78\"},{\"content\":{\"connectorIds\":[\"Out2\",\"Out1\"],\"side\":\"RIGHT\"},\"type\":\"ConnectorPlacement.EquallySpacedRectSide\",\"uuid\":\"c60e59f8-355a-4175-8fdf-4ec7731bebd5\"},{\"content\":{\"connectorIds\":[],\"side\":\"TOP\"},\"type\":\"ConnectorPlacement.EquallySpacedRectSide\",\"uuid\":\"9b883936-4238-4a8a-bb31-823c5677e2f1\"},{\"content\":{\"connectorIds\":[],\"side\":\"HIDDEN\"},\"type\":\"ConnectorPlacement.EquallySpacedRectSide\",\"uuid\":\"0dc2dc95-8f78-4c37-a0e8-9ab5748c0bf4\"}]},\"type\":\"ConnectorPlacement.EquallySpacedConnector\",\"uuid\":\"1656da2d-b85e-4414-b229-d0d15d73b339\"}],\"packageUris\":[\"http://schema.mathworks.com/mf0/Connector/R2020b\"],\"version\":\"1.0\"}"
  SPI_ISR : mbd_mpc574x_ec_toolbox/Communication Blocks/SPI Blocks/SPI_ISR  InstanceNumber=2  isr_lvl=0  role=Master  transfer_end=on  spi_upd=on
      settings: SourceProductName=NXP Model-Based Design Toolbox for MPC57xx MCUs
  SPI_ISR1 : mbd_mpc574x_ec_toolbox/Communication Blocks/SPI Blocks/SPI_ISR  InstanceNumber=1  isr_lvl=0  role=Master  transfer_end=on  spi_upd=on
      settings: SourceProductName=NXP Model-Based Design Toolbox for MPC57xx MCUs
  Subsystem : Subsystem
  Subsystem2 : Subsystem
  Subsystem3 : Subsystem
  input status : Subsystem
  mem copy read1 : Subsystem  TreatAsAtomicUnit=on
  send data spi1 : Subsystem
  write cmd eeprom1 : Subsystem  TreatAsAtomicUnit=on
  wires:
  Remote mc33978/2(send_spi()) -> Subsystem/Trigger
  Data Store Read/1 -> Driver TLE82453-3/1(FAULTN)
  Remote mc33978/1(out_data) -> Subsystem/1(send_spi())
  SPI_ISR1/1 -> Diagnostic1/Trigger
  SPI_ISR/1 -> input status/Trigger
  Driver TLE82453-3/2(out) -> Subsystem2/1(send_spi())
  Driver TLE82453-3/3(out2) -> Subsystem3/1(send_spi())
  Driver TLE82453-3/1(RESN) -> Data Store Write/1
  Data Store Read4/1 -> Driver TLE82453-3/3(setpoint)
  Driver TLE82453-3/4(send_spi()) -> Subsystem2/Trigger
  Data Store Read5/1 -> Driver TLE82453-3/2(RESET)
  Bit to Integer Converter1/1 -> Driver TLE82453-3/4(out_drv)
  Data Store Read3/1 -> Bit to Integer Converter1/1
  Driver TLE82453-3/5(send_spi2()) -> Subsystem3/Trigger
  EEPROM DRIVER1/5(mem_rd()) -> mem copy read1/Trigger
  Data Store Read9/1 -> EEPROM DRIVER1/2(wr_en)
  EEPROM DRIVER1/2(flag_idle) -> Data Store Write2/1
  Data Store Read8/1 -> EEPROM DRIVER1/3(in_data)
  EEPROM DRIVER1/1(out_data) -> send data spi1/1(out_data)
  EEPROM DRIVER1/4(send_spi()) -> send data spi1/Trigger
  Data Store Read11/1 -> EEPROM DRIVER1/1(adress)
  Data Store Read10/1 -> EEPROM DRIVER1/4(rd_en)
  EEPROM DRIVER1/3(wr_cmd()) -> write cmd eeprom1/Trigger

== system BCM2_4/Init System ==
  note: Иницилизация контроллера
  note: SPI INIT
  note: CAN INIT
  note: TLE824533 INIT
  CAN0_Config : mbd_mpc574x_ec_toolbox/Communication Blocks/CAN Blocks/FCAN_Config  Priority=1  can_instance=0  can_mode=Normal mode  can_max_num_mb=63  can_rx=PTB1: [CAN0_RX | CAN 0 Receive Pin]  can_tx=PTB0: [CAN0_TX | CAN 0 Transmit Pin]  show_adv_opts=on  can_clk_src=Peripheral clock  bitrate_to_time_seg=on  bitrate=250  sample_point=87.5  can_presdiv=18  can_propseg=7  can_pseg1=2  can_pseg2=1  can_rjw=2  cbt_bitrate=1000  cbt_sample_point=87.5  can_cbt_presdiv=1  can_cbt_propseg=6  can_cbt_pseg1=7  can_cbt_pseg2=7  can_cbt_rjw=3  can_fd_enable=off  can_payload=8  can_rxfifo_enable=off  can_fifo_id_filter_extended=off  can_fifo_id_filter_remote=off  can_num_id_filters=8  can_fifo_id_format=A  can_fifo_id_filter={'0x0', '0x0', '0x0', '0x0', '0x0', '0x0', '0x0', '0x0'}  can_pn_enable=off  can_wakeup_match=off  can_wakeup_timeout=off  can_timeout_en=off  can_match_timeout=1  can_multiple_matches_en=off  can_num_matches=1  can_idfilter_extendedid=off  can_idfilter_remoteframe=off  can_idfilter_type=Match exact  can_idfilter_id1=0  can_idfilter_id2=0  can_payloadfilter_enable=off  can_payloadfilter_dlclow=0  can_payloadfilter_dlchigh=0  can_payloadfilter_type=Match exact  can_payloadfilter_payload1_b0=0  can_payloadfilter_payload1_b1=0  can_payloadfilter_payload1_b2=0  can_payloadfilter_payload1_b3=0  can_payloadfilter_payload1_b4=0  can_payloadfilter_payload1_b5=0  can_payloadfilter_payload1_b6=0  can_payloadfilter_payload1_b7=0  can_payloadfilter_payload2_b0=0  can_payloadfilter_payload2_b1=0  can_payloadfilter_payload2_b2=0  can_payloadfilter_payload2_b3=0  can_payloadfilter_payload2_b4=0  can_payloadfilter_payload2_b5=0  can_payloadfilter_payload2_b6=0  can_payloadfilter_payload2_b7=0
  CAN1_Config : mbd_mpc574x_ec_toolbox/Communication Blocks/CAN Blocks/FCAN_Config  Priority=4  can_instance=1  can_mode=Normal mode  can_max_num_mb=63  can_rx=PTA15: [CAN1_RX | CAN 1 Receive Pin]  can_tx=PTA14: [CAN1_TX | CAN 1 Transmit Pin]  show_adv_opts=on  can_clk_src=Peripheral clock  bitrate_to_time_seg=on  bitrate=250  sample_point=87.5  can_presdiv=18  can_propseg=7  can_pseg1=2  can_pseg2=1  can_rjw=2  cbt_bitrate=1000  cbt_sample_point=87.5  can_cbt_presdiv=1  can_cbt_propseg=6  can_cbt_pseg1=7  can_cbt_pseg2=7  can_cbt_rjw=3  can_fd_enable=off  can_payload=8  can_rxfifo_enable=off  can_fifo_id_filter_extended=off  can_fifo_id_filter_remote=off  can_num_id_filters=8  can_fifo_id_format=A  can_fifo_id_filter={'0x0', '0x0', '0x0', '0x0', '0x0', '0x0', '0x0', '0x0'}  can_pn_enable=off  can_wakeup_match=off  can_wakeup_timeout=off  can_timeout_en=off  can_match_timeout=1  can_multiple_matches_en=off  can_num_matches=1  can_idfilter_extendedid=off  can_idfilter_remoteframe=off  can_idfilter_type=Match exact  can_idfilter_id1=0  can_idfilter_id2=0  can_payloadfilter_enable=off  can_payloadfilter_dlclow=0  can_payloadfilter_dlchigh=0  can_payloadfilter_type=Match exact  can_payloadfilter_payload1_b0=0  can_payloadfilter_payload1_b1=0  can_payloadfilter_payload1_b2=0  can_payloadfilter_payload1_b3=0  can_payloadfilter_payload1_b4=0  can_payloadfilter_payload1_b5=0  can_payloadfilter_payload1_b6=0  can_payloadfilter_payload1_b7=0  can_payloadfilter_payload2_b0=0  can_payloadfilter_payload2_b1=0  can_payloadfilter_payload2_b2=0  can_payloadfilter_payload2_b3=0  can_payloadfilter_payload2_b4=0  can_payloadfilter_payload2_b5=0  can_payloadfilter_payload2_b6=0  can_payloadfilter_payload2_b7=0
      settings: SourceProductName=NXP Model-Based Design Toolbox for MPC57xx MCUs
  CAN2_Config : mbd_mpc574x_ec_toolbox/Communication Blocks/CAN Blocks/FCAN_Config  Priority=4  can_instance=2  can_mode=Normal mode  can_max_num_mb=63  can_rx=PTF15: [CAN2_RX | CAN2 RXD]  can_tx=PTF14: [CAN2_TX | CAN 2 Transmit Pin]  show_adv_opts=on  can_clk_src=Peripheral clock  bitrate_to_time_seg=on  bitrate=250  sample_point=87.5  can_presdiv=18  can_propseg=7  can_pseg1=2  can_pseg2=1  can_rjw=2  cbt_bitrate=1000  cbt_sample_point=87.5  can_cbt_presdiv=1  can_cbt_propseg=6  can_cbt_pseg1=7  can_cbt_pseg2=7  can_cbt_rjw=3  can_fd_enable=off  can_payload=8  can_rxfifo_enable=off  can_fifo_id_filter_extended=off  can_fifo_id_filter_remote=off  can_num_id_filters=8  can_fifo_id_format=A  can_fifo_id_filter={'0x0', '0x0', '0x0', '0x0', '0x0', '0x0', '0x0', '0x0'}  can_pn_enable=off  can_wakeup_match=off  can_wakeup_timeout=off  can_timeout_en=off  can_match_timeout=1  can_multiple_matches_en=off  can_num_matches=1  can_idfilter_extendedid=off  can_idfilter_remoteframe=off  can_idfilter_type=Match exact  can_idfilter_id1=0  can_idfilter_id2=0  can_payloadfilter_enable=off  can_payloadfilter_dlclow=0  can_payloadfilter_dlchigh=0  can_payloadfilter_type=Match exact  can_payloadfilter_payload1_b0=0  can_payloadfilter_payload1_b1=0  can_payloadfilter_payload1_b2=0  can_payloadfilter_payload1_b3=0  can_payloadfilter_payload1_b4=0  can_payloadfilter_payload1_b5=0  can_payloadfilter_payload1_b6=0  can_payloadfilter_payload1_b7=0  can_payloadfilter_payload2_b0=0  can_payloadfilter_payload2_b1=0  can_payloadfilter_payload2_b2=0  can_payloadfilter_payload2_b3=0  can_payloadfilter_payload2_b4=0  can_payloadfilter_payload2_b5=0  can_payloadfilter_payload2_b6=0  can_payloadfilter_payload2_b7=0
      settings: SourceProductName=NXP Model-Based Design Toolbox for MPC57xx MCUs
  Constant1 : Constant  Value=0.5  OutDataTypeStr=single  SampleTime=-1
  Data Store Read2 : DataStoreRead  DataStoreName=RESN  IndexOptions=Index vector (dialog)  Indices=1  OutputSizes=1
  Data Store Write2 : DataStoreWrite  DataStoreName=FAULTN  IndexOptions=Index vector (dialog)  Indices=1  OutputSizes=1
  Digital_Input : mbd_mpc574x_ec_toolbox/GPIO Blocks/Digital_Input  gpio_pin=PTE7: [SIUL2_GPI71 | General Purpose IO PE[7]]  pull_resistor=Pullup
      settings: SourceProductName=NXP Model-Based Design Toolbox for MPC57xx MCUs
  Digital_Output1 : mbd_mpc574x_ec_toolbox/GPIO Blocks/Digital_Output  gpio_pin=PTB6: [SIUL2_GPIO22 | General Purpose IO PB[6]]  gpio_drive_strength=Disabled
      settings: SourceProductName=NXP Model-Based Design Toolbox for MPC57xx MCUs
  FTM_PWM_Config : mbd_mpc574x_ec_toolbox/Motor Control Blocks/FlexPWM Blocks/FlexPWM_Config  Priority=1  pwmModule=0  pwmSubmodule=0  pwmMode=Edge aligned PWM  pwmPair=Independent  pwmCompSource=PWM45  pwmCounterInit=Local sync (PWMX)  pwmClockSource=Peripheral clock  pwmUnits=Hz  pwmFrequency=8000000  pwmPeriod=10  pwmPrescaler=Divide by 1  pwmDtUnits=Nanoseconds  pwmDtNs=500  pwmDtTicks=40  pwmReloadLogic=Half & Full Cycle  pwmReloadFrequency=Every 1 PWM opportunity  pwmTriggeringSignal=Local force signal  pwmDutyCycleOutSim=off  pwmStartAfterInit=on  pwmShowAdvOpts=off  pwmPinA=PTA11: [PWM0_A0 | FlexPWM_0 Channel A Input/Output 0]  pwmPinB=None  pwmPolarityA=off  pwmPolarityB=off  pwmAInitialVal=0.5  pwmBInitialVal=0.5  pwmAShift=0  pwmBShift=0  trgReloadISR=off  trgVal0=off  trgVal1=off  trgVal2=off  trgVal3=off  trgVal4=off  trgVal5=off  trgReloadErrorISR=off  pwmPinFault=None  PwmFaultEnISR=off  pwmFaultEnA=off  pwmFaultEnB=off
      settings: SourceProductName=NXP Model-Based Design Toolbox for MPC57xx MCUs
  FreeMaster_Config : mbd_mpc574x_ec_toolbox/Utility Blocks/FreeMaster_Config  Priority=2  interface=Serial0  baudrate=115200  rxd=PTB3: [LIN0_RX | LIN 0 Receive Pin]  txd=PTB2: [LIN0_TX | LINFlexD 0 Transmit Pin]  mode=Short Interrupt  isr_prio=1  show_adv_opts=on  use_scope=on  max_scope_vars=8  use_recorder=on  max_rec_vars=8  rec_buff_size=1024  rec_timebase=0 seconds  comm_buffer_size_auto=on  comm_buffer_size=255  comm_rqueue_size_default=on  comm_rqueue_size=32
      settings: SourceProductName=NXP Model-Based Design Toolbox for MPC57xx MCUs
  MBD_MPC574x_Config_Information : mbd_mpc574x_ec_toolbox/MBD_MPC574x_Config_Information  Priority=0  disp_str=|  config_params=[]  mcu_target_name=MPC5744P  mcu_target_package=144-LQFP  mcu_target_sram_size=384KB  mcu_system_clock_freq=200  mcu_xtal_freq=40  mcu_step_timer=PIT Channel 0  mcu_step_priority=1  ds_import_enable=on  target_compiler=S32 Design Studio  target_memory=FLASH  s32ds_target_compile_opts=-g3 -mbig -mvle -O1 -mregnames -mlsp -specs=ewl_c9x.specs -mhard-float -Wall -c -std=c99 -fdata-sections -ffunction-sections -funsigned-char -fmessage-length=0 -nostdinc -fno-jump-tables  s32ds_target_assemble_opts=-g3 -mbig -mvle -mregnames  s32ds_target_link_opts=-Xlinker --gc-sections -mhard-float  s32ds_target_default_lcf=on  s32ds_target_user_lcf=MPC5744P_flash.ld  ghs_target_compile_opts=-preprocess_assembly_files -g -dwarf2 -noSPE -filetype.c  ghs_target_assemble_opts=-preprocess_assembly_files -g -dwarf2 -e _start_core -srec -filetype.assembly  ghs_target_default_lcf=on  ghs_target_user_lcf=MPC5744P_flash.ld  diab_target_compile_opts=-@E+err.log -c -g -Xenum-is-best -Xlint -Xnested-interrupts -Xdebug-local-cie -Xclib-optim-off -Xc-new  diab_target_assemble_opts=-@E+err.log -l -g  diab_target_link_opts=-@E+err.log -Ws -m6 -lc -lm  diab_target_default_lcf=on  diab_target_user_lcf=MPC5744P_flash.dld  pil_download_enable=off  rbl_download_enable=on  rbl_start_delay=2000  rbl_restart_request=on  rbl_com_port=Custom  rbl_com_port_custom=COM6  pil_download_rate=115200  pil_interface=Serial 0  pil_rx=PTB3: [LIN0_RX | LIN 0 Receive Pin]  pil_tx=PTB2: [LIN0_TX | LINFlexD 0 Transmit Pin]  rbl_def_password=on  rbl_password=0xFEEDFACECAFEBEEF  rbl_manual_len_size=off  rbl_start_address=0  rbl_code_size=0  ADC_PcrCheckEnDis=on  FlexPWM_PcrCheckEnDis=on  CTU_PcrCheckEnDis=on  SWG_PcrCheckEnDis=on  eTimer_PcrCheckEnDis=on  EQADC_PcrCheckEnDis=on  eMIOS_PcrCheckEnDis=on  FlexCAN_PcrCheckEnDis=on  I2C_PcrCheckEnDis=on  MCAN_PcrCheckEnDis=on  SPI_PcrCheckEnDis=on  UART_PcrCheckEnDis=on  GPIO_OutputPcrCheckEnDis=on  GPIO_InputPcrCheckEnDis=on  eDMA_PcrCheckEnDis=on  PIT_PcrCheckEnDis=on  AMMCLIB_PcrCheckEnDis=on  FM_PcrCheckEnDis=on  Profiler_PcrCheckEnDis=on  ModelRef_PcrCheckEnDis=on  ModelPinCheck_PcrCheckEnDis=on
      | System Clock : 200 MHz
      | Target : MPC5744P
      | Package : 144LQFP
      | XTAL Freq : 40 MHz
      | Compiler : S32 Design Studio
      | Target Type : FLASH
      | Global Interrupt Priority : 8
      | System Tick Interrupt Priority : 12
      | Freemaster : None;
      | Download Code after build : off
  SPI_Config EEPROM : mbd_mpc574x_ec_toolbox/Communication Blocks/SPI Blocks/SPI_Config  InstanceNumber=3  Role=Master  BaudRate=1000000  ShowAdvanced=on  sin=PTD14: [DSPI3_SIN | DSPI 3 Serial Data Input]  sout=PTD5: [DSPI3_SOUT | DSPI 3 Serial Data Out]  sck=PTD6: [DSPI3_SCK | DSPI 3 Input/Output Serial Clock]  pcs0=PTF5: [DSPI3_CS0 | DSPI 3 Peripheral Chip Select 0]  pcs1=None  pcs2=None  pcs3=None  pcs4=None  pcs5=None  pcs6=None  pcs7=None  CPHA=DSPI_CLOCK_PHASE_2ND_EDGE  CPOL=DSPI_ACTIVE_LOW  BitOrder=MSB first  TransferSize=8  WhichPCS=0  PCSPol=DSPI_ACTIVE_LOW  ContinuousTransfer=on
  SPI_Config MC33978 : mbd_mpc574x_ec_toolbox/Communication Blocks/SPI Blocks/SPI_Config  InstanceNumber=2  Role=Master  BaudRate=1000000  ShowAdvanced=on  sin=PTA2: [DSPI2_SIN | DSPI 2 Serial Data Input]  sout=PTA1: [DSPI2_SOUT | DSPI 2 Serial Data Out]  sck=PTA0: [DSPI2_SCK | DSPI 2 Input/Output Serial Clock]  pcs0=None  pcs1=None  pcs2=None  pcs3=PTG10: [DSPI2_CS3 | DSPI 2 Peripheral Chip Select 3]  pcs4=None  pcs5=None  pcs6=None  pcs7=None  CPHA=DSPI_CLOCK_PHASE_1ST_EDGE  CPOL=DSPI_ACTIVE_HIGH  BitOrder=MSB first  TransferSize=8  WhichPCS=0  PCSPol=DSPI_ACTIVE_LOW  ContinuousTransfer=on
      settings: SourceProductName=NXP Model-Based Design Toolbox for MPC57xx MCUs
  SPI_Config output driver : mbd_mpc574x_ec_toolbox/Communication Blocks/SPI Blocks/SPI_Config  InstanceNumber=1  Role=Master  BaudRate=1000000  ShowAdvanced=on  sin=PTA8: [DSPI1_SIN | DSPI 1 Serial Data Input]  sout=PTA7: [DSPI1_SOUT | DSPI 1 Serial Data Out]  sck=PTA6: [DSPI1_SCK | DSPI 1 Input/Output Serial Clock]  pcs0=PTA5: [DSPI1_CS0 | DSPI 1 Peripheral Chip Select 0]  pcs1=PTG2: [DSPI1_CS1 | DSPI 1 Peripheral Chip Select 1]  pcs2=None  pcs3=None  pcs4=None  pcs5=None  pcs6=None  pcs7=None  CPHA=DSPI_CLOCK_PHASE_2ND_EDGE  CPOL=DSPI_ACTIVE_HIGH  BitOrder=MSB first  TransferSize=8  WhichPCS=0  PCSPol=DSPI_ACTIVE_LOW  ContinuousTransfer=on
      settings: SourceProductName=NXP Model-Based Design Toolbox for MPC57xx MCUs
  Начальная иницилизация : Subsystem  TreatAsAtomicUnit=on
  wires:
  Digital_Input/1 -> Data Store Write2/1
  Data Store Read2/1 -> Digital_Output1/1
  Constant1/1 -> FTM_PWM_Config/1

== system BCM2_4/retarder/work.ret_on.table ==
  Action Port : ActionPort
      settings: CopyFcn=Stateflow.SLINSF.SimulinkMan.removeBlockPreDeleteFcn  PreDeleteFcn=Stateflow.SLINSF.SimulinkMan.unsafePredeleteFcn
  2-D Lookup Table : Lookup_n-D  BreakpointsForDimension1=[200,400,600,800,1000,1200,1400,1600,1800,2000,2200,2400,2600,2800]  BreakpointsForDimension2=[0,250,500,750,1000,1250,1500,1750,2000,2250,2500,2750,3000,3250,3500,3750,4000]  Table=reshape([0,0,0,0,0,0,0,0,0,0,0,0,0,0,231,158,138.3,120,105,95,85,70,60,60,52.5,45,37.5,30,462.8,316.6,276.7,240,210,185,170,140,120,120,105,90,75,60,1019.9,761.9,535.1,389.3,334.6,291,255,210,180,180,157.9,135.8,113.7,91.6,1200,1131,912.3,704.6,568.1,442.6,348.3,285,252.8,251.8,250.9,250.1,249.2,238.4,1200,1200,1093.5,893.8,715.2,567.6,471,415.5,371,360.8,359.9,329,318.1,337.2,1200,1200,1199.4,967.1,800.9,651.1,548.2,482.2,432.6,429.1,424.3,389.6,384.8,380.1,1200,1200,1190.2,1034.3,871.8,691.8,593.6,506.4,469.6,472.9,465.1,437.2,429.4,411.6,1200,1200,1200,1144.7,973.3,815.4,700.7,619.2,570.2,562.9,545.9,538.9,531.9,524.9,1200,1200,1200,1200,1175.5,1027.5,910.4,824.9,771.8,751,732.3,713.6,694.9,676.2,1200,1200,1200,1200,1200,1003.5,956.9,926.5,901,877.3,866.6,860.6,854.6,838.6,1200,1200,1200,1200,1200,1200,1200,1035.3,928.8,888.9,872.9,857,841,825,1200,1200,1200,1200,1200,1200,1200,1156.1,975.3,861.3,814.2,807.5,800.8,794.1,1200,1200,1200,1200,1200,1200,1200,1200,1014.4,856.5,745.3,740.9,663.3,662.4,1200,1200,1200,1200,1200,1200,1200,1200,1197.2,957,757.6,688.8,570.6,443,1200,1200,1200,1200,1200,1200,1200,1200,1200,1200,822.5,671.3,508.8,345.3,1200,1200,1200,1200,1200,1200,1200,1200,1200,1200,915.2,670.6,514.4,316.9],14,17)  ExtrapMethod=Clip  InternalRulePriority=Speed  RndMeth=Simplest  InputSameDT=on
      settings: InputPortMap=u0,u1
  Data Store Read : DataStoreRead  DataStoreName=ret  DataStoreElements=ret.AT_out#ret.M  IndexOptions=Index vector (dialog)  Indices=1  OutputSizes=1
  Data Store Write : DataStoreWrite  DataStoreName=Ivalve  DataStoreElements=Ivalve(2)  IndexOptions=Index vector (dialog)  Indices=1  OutputSizes=1
  Saturation : Saturate  UpperLimit=1200  LowerLimit=0
  wires:
  Data Store Read/1 -> 2-D Lookup Table/1
  Data Store Read/2 -> 2-D Lookup Table/2
  2-D Lookup Table/1 -> Saturation/1
  Saturation/1 -> Data Store Write/1

== system BCM2_4/tank ==
  In_tank1 : Inport
  In_tank2 : Inport  Port=2
  In_tank3 : Inport  Port=3
  Add : Sum
  Add1 : Sum
  Add2 : Sum
  Band-Limited White Noise2 : simulink/Sources/Band-Limited White Noise  Cov=[2 2 2]  Ts=0.2  seed=[23341 51748 18375]
  Demux : Demux  Outputs=3
  Saturation : Saturate  UpperLimit=330  LowerLimit=0
  Saturation1 : Saturate  UpperLimit=330  LowerLimit=0
  Saturation2 : Saturate  UpperLimit=200  LowerLimit=0
  Switch : Switch  Criteria=u2 > Threshold  Threshold=1
  Switch1 : Switch  Criteria=u2 > Threshold  Threshold=1
  Switch2 : Switch  Criteria=u2 > Threshold  Threshold=1
  Out_tank1 : Outport
  Out_tank2 : Outport  Port=2
  Out_tank3 : Outport  Port=3
  wires:
  Add2/1 -> Switch2/1
  Add1/1 -> Switch1/1
  Add/1 -> Switch/1
  In_tank1/1 -> Switch/2, Switch/3, Add/1
  In_tank2/1 -> Add1/1, Switch1/3, Switch1/2
  In_tank3/1 -> Switch2/2, Switch2/3, Add2/1
  Saturation/1 -> Out_tank1/1
  Saturation1/1 -> Out_tank2/1
  Saturation2/1 -> Out_tank3/1
  Switch/1 -> Saturation/1
  Switch1/1 -> Saturation1/1
  Switch2/1 -> Saturation2/1
  Band-Limited White Noise2/1 -> Demux/1
  Demux/1 -> Add/2
  Demux/2 -> Add1/2
  Demux/3 -> Add2/2

== system BCM2_4/Беспроводной руль ==
  Compare To Constant : simulink/Logic and Bit Operations/Compare To Constant  relop===  const=1  OutDataTypeStr=boolean
  Compare To Constant1 : simulink/Logic and Bit Operations/Compare To Constant  relop===  const=2  OutDataTypeStr=boolean
  Compare To Constant2 : simulink/Logic and Bit Operations/Compare To Constant  relop===  const=3  OutDataTypeStr=boolean
  Compare To Constant3 : simulink/Logic and Bit Operations/Compare To Constant  relop===  const=4  OutDataTypeStr=boolean
  Compare To Constant4 : simulink/Logic and Bit Operations/Compare To Constant  relop===  const=5  OutDataTypeStr=boolean
  Compare To Constant5 : simulink/Logic and Bit Operations/Compare To Constant  relop===  const=6  OutDataTypeStr=boolean
  Data Store Read4 : DataStoreRead  DataStoreName=CAN_rec  DataStoreElements=CAN_rec.wireless_chan  IndexOptions=Index vector (dialog)  Indices=1  OutputSizes=1
  Data Store Write2 : DataStoreWrite  DataStoreName=CAN_trm  DataStoreElements=CAN_trm.wCCset#CAN_trm.wCCresume#CAN_trm.wCCacc#CAN_trm.wCCcoast#CAN_trm.wPilotPageP#CAN_trm.wPilotPageM  IndexOptions=Index vector (dialog)  Indices=1  OutputSizes=1
  wires:
  Data Store Read4/1 -> Compare To Constant3/1, Compare To Constant4/1, Compare To Constant5/1, Compare To Constant1/1, Compare To Constant/1, Compare To Constant2/1
  Compare To Constant/1 -> Data Store Write2/1
  Compare To Constant1/1 -> Data Store Write2/2
  Compare To Constant2/1 -> Data Store Write2/3
  Compare To Constant3/1 -> Data Store Write2/4
  Compare To Constant4/1 -> Data Store Write2/5
  Compare To Constant5/1 -> Data Store Write2/6

== system BCM2_4/Подогрев стекла ==
  Enable : EnablePort  StatesWhenEnabling=reset
  Data Type Conversion : DataTypeConversion  OutDataTypeStr=boolean
  Discrete Pulse Generator : DiscretePulseGenerator  Period=540  PulseWidth=360
  Out1 : Outport  OutputWhenDisabled=reset  InitialOutput=0
  wires:
  Discrete Pulse Generator/1 -> Data Type Conversion/1
  Data Type Conversion/1 -> Out1/1

== system BCM2_4/Расход топлива ==
  Add : Sum  Inputs=+++
  Data Store Read4 : DataStoreRead  DataStoreName=CAN_rec  DataStoreElements=CAN_rec.total_dist  IndexOptions=Index vector (dialog)  Indices=1  OutputSizes=1
  Data Store Read5 : DataStoreRead  DataStoreName=CAN_rec  DataStoreElements=CAN_rec.FuelTank1#CAN_rec.FuelTank2#CAN_rec.FuelTank3  IndexOptions=Index vector (dialog)  Indices=1  OutputSizes=1
  Data Store Write2 : DataStoreWrite  DataStoreName=CAN_trm  DataStoreElements=CAN_trm.rashod  IndexOptions=Index vector (dialog)  Indices=1  OutputSizes=1
  Data Type Conversion1 : DataTypeConversion  OutDataTypeStr=uint32
  Data Type Conversion2 : DataTypeConversion  OutDataTypeStr=uint16
  Расход топлива : Stateflow chart  TreatAsAtomicUnit=on
  wires:
  Data Store Read5/3 -> Add/3
  Data Store Read5/1 -> Add/1
  Add/1 -> Расход топлива/2(fuel)
  [in_trip] -> Расход топлива/1(trip)
  Расход топлива/1(r) -> Data Type Conversion2/1
  Data Store Read4/1 -> Data Type Conversion1/1
  Data Store Read5/2 -> Add/2
  Data Type Conversion1/1 -> Расход топлива/3(dist)
  Data Type Conversion2/1 -> Data Store Write2/1
